simulink model "Sistema_Automatizado"  (R2026a)
settings: Solver=VariableStepAuto  StopTime=12

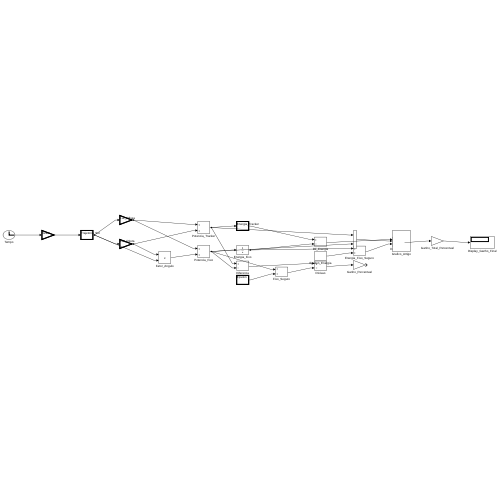
[thumbnail: Simulink's stored preview of the top-level diagram]
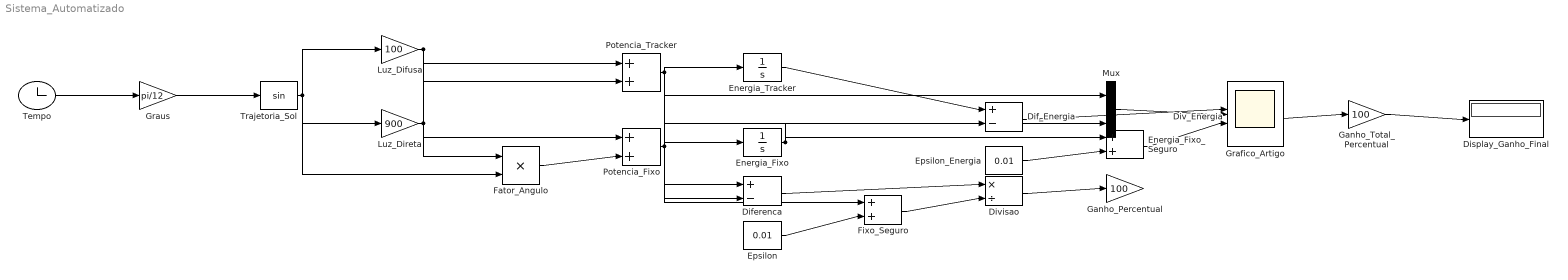
== system Sistema_Automatizado ==
  Dif_Energia : Sum  Inputs=+-
  Diferenca : Sum  Inputs=+-
  Display_Ganho_Final : Display
  Div_Energia : Product  Inputs=*/
  Divisao : Product  Inputs=*/
  Energia_Fixo : Integrator
  Energia_Fixo_Seguro : Sum
  Energia_Tracker : Integrator
  Epsilon : Constant  Value=0.01
  Epsilon_Energia : Constant  Value=0.01
  Fator_Angulo : Product
  Fixo_Seguro : Sum
  Ganho_Percentual : Gain  Gain=100
  Ganho_Total_Percentual : Gain  Gain=100
  Grafico_Artigo : Scope
  Graus : Gain  Gain=pi/12
  Luz_Difusa : Gain  Gain=100
  Luz_Direta : Gain  Gain=900
  Mux : Mux  Inputs=2
  Potencia_Fixo : Sum
  Potencia_Tracker : Sum
  Tempo : Clock
  Trajetoria_Sol : Trigonometry
  wires:
  Tempo/1 -> Graus/1
  Graus/1 -> Trajetoria_Sol/1
  Trajetoria_Sol/1 -> Luz_Difusa/1, Luz_Direta/1, Fator_Angulo/2
  Luz_Difusa/1 -> Potencia_Tracker/1, Potencia_Fixo/1
  Luz_Direta/1 -> Potencia_Tracker/2, Fator_Angulo/1
  Fator_Angulo/1 -> Potencia_Fixo/2
  Potencia_Tracker/1 -> Diferenca/1, Energia_Tracker/1, Mux/1
  Potencia_Fixo/1 -> Diferenca/2, Fixo_Seguro/1, Energia_Fixo/1, Mux/2
  Epsilon/1 -> Fixo_Seguro/2
  Diferenca/1 -> Divisao/1
  Fixo_Seguro/1 -> Divisao/2
  Divisao/1 -> Ganho_Percentual/1
  Energia_Tracker/1 -> Dif_Energia/1
  Energia_Fixo/1 -> Dif_Energia/2, Energia_Fixo_Seguro/1
  Epsilon_Energia/1 -> Energia_Fixo_Seguro/2
  Dif_Energia/1 -> Div_Energia/1
  Energia_Fixo_Seguro/1 -> Div_Energia/2
  Div_Energia/1 -> Ganho_Total_Percentual/1
  Ganho_Total_Percentual/1 -> Display_Ganho_Final/1
  Mux/1 -> Grafico_Artigo/1
